simulink model "power_OLTCregtransformer"  (Simulink 6.0)
settings: Solver=ode23tb  StartTime=0.0  StopTime=120  MaxStep=1/60  RelTol=1e-4  AbsTol=1e-3
libraries: powerlib x75, powerlib_extras x18, simulink_extras x1
(part 3 of 3)

== system power_OLTCregtransformer/Three-Phase OLTC Regulating Transformer (Phasor Type)/Z & Voltage Ratio/Z Tap on winding 2 ==
  note: Tap changer on winding 2:
      | Z = Zw1  + Zw2*1/(1+NdU)^2 +  Ztmax*N*Nmax*(dU)^2/(1+NdU)^2
      | N1/N2= 1/(1+NdU)
      |
      | where :
      | Zw1   =  impedance of winding 1 (pu based on Pnom and V1nom)
      | Zw2   =  impedance of winding 2 (pu based on Pnom and V2nom)
      | Ztmax = impedance of tapped winding at maximum tap (Nmax)     (pu  based on  Pnom & Nmax*dU)
      | Zt =  impedance of tapped winding at tap N
      |      = Ztmax*N/Nmax*(Nmax.dU)^2 = Ztmax*N*Nmax*(dU)^2             (pu based on Pnom and V2nom)
  N : Inport  Port=1  LatchInput=off
  dU : Inport  Port=2  LatchInput=off
  Zw1 : Inport  Port=3  LatchInput=off
  Zw2 : Inport  Port=4  LatchInput=off
  Ztmax : Inport  Port=5  LatchInput=off
  Nmax : Inport  Port=6  LatchInput=off
  Enable : EnablePort
  Math Function1 : Math  Operator=reciprocal  SaturateOnIntegerOverflow=on
  Math Function2 : Math  Operator=square  SaturateOnIntegerOverflow=on
  Math Function5 : Math  Operator=square  SaturateOnIntegerOverflow=on
  Product1 : Product  SaturateOnIntegerOverflow=on
  Product2 : Product  Inputs=*/  SaturateOnIntegerOverflow=on
  Product3 : Product  Inputs=****  SaturateOnIntegerOverflow=on
  Product6 : Product  Inputs=*/  SaturateOnIntegerOverflow=on
  Psi1 : Constant
  Sum1 : Sum  Inputs=+++  SaturateOnIntegerOverflow=on
  Sum2 : Sum  SaturateOnIntegerOverflow=on
  Z : Outport
  N1/N2 : Outport  Port=2
  wires:
  Math Function1/1 -> N1/N2/1
  Product6/1 -> Sum1/1
  Product3/1 -> Product6/1  "Zt = Ztmax*N*Nmax*(dU)^2"
  Math Function2/1 -> Product6/2, Product2/2
  Zw2/1 -> Product2/1
  Product2/1 -> Sum1/2
  Sum1/1 -> Z/1
  Zw1/1 -> Sum1/3
  Psi1/1 -> Sum2/2
  Sum2/1 -> Math Function1/1, Math Function2/1  "1+NdU"
  N/1 -> Product1/1, Product3/3
  dU/1 -> Math Function5/1, Product1/2
  Product1/1 -> Sum2/1  "NdU"
  Ztmax/1 -> Product3/1
  Nmax/1 -> Product3/2
  Math Function5/1 -> Product3/4

== system power_OLTCregtransformer/Three-Phase OLTC Regulating Transformer/ OLTC Control/Monostable/Edge Detector ==
  note: Edge or Slope Detector
  note: Silvano Casoria
      | Power System Simulation Laboratory
      | IREQ, Hydro-Quebec
  In : Inport  Port=1  LatchInput=off
  Constant1 : Constant  Value=model
  Demux : Demux  Outputs=2
  Logical Operator1 : Logic  Operator=OR
  Memory : Memory  X0=ic  InheritSampleTime=on
  Multiport Switch : MultiPortSwitch  Inputs=3  SaturateOnIntegerOverflow=on
  NEGATIVE Edge : Subsystem  AncestorBlock=extra_sc/Edge/POSITIVE Edge  TreatAsAtomicUnit=on
  POSITIVE Edge : Subsystem  AncestorBlock=extra_sc/Delay_discrete/OFF Delay  TreatAsAtomicUnit=on
  either edge : Constant  Value=[1 1]
  neg. edge : Constant  Value=[0 1]
  pos. edge : Constant  Value=[1 0]
  Out : Outport
  wires:
  either edge/1 -> Multiport Switch/4
  Demux/2 -> NEGATIVE Edge/Enable
  Demux/1 -> POSITIVE Edge/Enable
  Multiport Switch/1 -> Demux/1
  Constant1/1 -> Multiport Switch/1
  neg. edge/1 -> Multiport Switch/3
  pos. edge/1 -> Multiport Switch/2
  In/1 -> Memory/1, NEGATIVE Edge/1(IN), POSITIVE Edge/1(IN)
  Memory/1 -> NEGATIVE Edge/2(IN previous), POSITIVE Edge/2(IN previous)
  POSITIVE Edge/1(OUT) -> Logical Operator1/1
  NEGATIVE Edge/1(OUT) -> Logical Operator1/2
  Logical Operator1/1 -> Out/1

== system power_OLTCregtransformer/Three-Phase OLTC Regulating Transformer/ OLTC Control/Tap Changer Control/Determine tap positon ==
  NewTap : Inport  Port=1  LatchInput=off
  Trigger : TriggerPort
  Memory : Memory  Orientation=left  X0=InitialPosition  InheritSampleTime=on
  Saturation : Saturate  UpperLimit=MinMaxTap(2)  LowerLimit=MinMaxTap(1)
  Sum : Sum  Inputs=|++  SaturateOnIntegerOverflow=on
  TapNo : Outport  InitialOutput=InitialPosition
  wires:
  NewTap/1 -> Sum/1
  Sum/1 -> Saturation/1
  Memory/1 -> Sum/2
  Saturation/1 -> TapNo/1, Memory/1

== system power_OLTCregtransformer/Three-Phase OLTC Regulating Transformer (Phasor Type)/ Currents /dq0 model of 3-ph RL branch/Negative-sequence dq0 model of a 3-phase series R-L branch ==
  note: Using Laplace transform and per unit (pu) quantities :
  note: d-q axis model of a 3-phase series R-L branch
  note: Id = [ w / ( L * s ) ] * [ Vd1 - Vd2 - ( R * Id ) + ( L * Iq ) ]
  note: Iq = [ w / ( L * s ) ] * [ Vq1 - Vq2 - ( R * Iq ) - ( L * Id ) ]
  note: where w = 2*pi*Fnom (Hz)
  note: Vd1 - Vd2 = [ R * Id ] - [ L* w * Iq ] + [ L * d/dt (Id) ]
  note: o--------| R |---| L |-------o
  note: V1
  note: V2
  note: I --->
  note: ==========================================================================================
  note: Vq1 - Vq2 = [ R * Iq ] + [ L* w * Id ] + [ L * d/dt (Iq) ]
  note: where w = 2*pi*Fnom (Hz)
  Vdq1 : Inport  Port=1  LatchInput=off
  Vdq2 : Inport  Port=2  LatchInput=off
  R_L : Inport  Port=3  LatchInput=off
  Demux3 : Demux  Outputs=2
  Integrator : Integrator
  Product : Product  SaturateOnIntegerOverflow=on
  Product1 : Product  SaturateOnIntegerOverflow=on
  Product2 : Product  Inputs=*/  SaturateOnIntegerOverflow=on
  R_choke2 : Gain  Gain=[1 -1]  SaturateOnIntegerOverflow=on
  R_choke3 : Gain  Gain=w  SaturateOnIntegerOverflow=on
  Selector : Selector  Elements=[2 1]  InputPortWidth=2
  Sum : Sum  Inputs=+--+  SaturateOnIntegerOverflow=on
  idIq : Outport
  wires:
  Vdq1/1 -> Sum/1
  Vdq2/1 -> Sum/2
  Product/1 -> Sum/3
  R_choke2/1 -> Sum/4
  Product1/1 -> R_choke2/1
  Sum/1 -> R_choke3/1
  Integrator/1 -> idIq/1, Selector/1, Product/1
  Selector/1 -> Product1/1
  R_choke3/1 -> Product2/1
  Product2/1 -> Integrator/1
  R_L/1 -> Demux3/1
  Demux3/2 -> Product2/2, Product1/2
  Demux3/1 -> Product/2

== system power_OLTCregtransformer/Three-Phase OLTC Regulating Transformer (Phasor Type)/ Currents /dq0 model of 3-ph RL branch/Positive-sequence dq0 model of a 3-phase series R-L branch ==
  note: where w = 2*pi*Fnom (Hz)
  note: Vq1 - Vq2 = [ R * Iq ] + [ L* w * Id ] + [ L * d/dt (Iq) ]
  note: ==========================================================================================
  note: I --->
  note: V2
  note: V1
  note: o--------| R |---| L |-------o
  note: Vd1 - Vd2 = [ R * Id ] - [ L* w * Iq ] + [ L * d/dt (Id) ]
  note: where w = 2*pi*Fnom (Hz)
  note: Iq = [ w / ( L * s ) ] * [ Vq1 - Vq2 - ( R * Iq ) - ( L * Id ) ]
  note: Id = [ w / ( L * s ) ] * [ Vd1 - Vd2 - ( R * Id ) + ( L * Iq ) ]
  note: d-q axis model of a 3-phase series R-L branch
  note: Using Laplace transform and per unit (pu) quantities :
  Vdq1 : Inport  Port=1  LatchInput=off
  Vdq2 : Inport  Port=2  LatchInput=off
  R_L : Inport  Port=3  LatchInput=off
  Demux3 : Demux  Outputs=2
  Integrator : Integrator  InitialCondition="[I21_init_real   I21_init_imag]"
  Product : Product  SaturateOnIntegerOverflow=on
  Product1 : Product  SaturateOnIntegerOverflow=on
  Product2 : Product  Inputs=*/  SaturateOnIntegerOverflow=on
  R_choke2 : Gain  Gain=[1 -1]  SaturateOnIntegerOverflow=on
  R_choke3 : Gain  Gain=w  SaturateOnIntegerOverflow=on
  Selector : Selector  Elements=[2 1]  InputPortWidth=2
  Sum : Sum  Inputs=+--+  SaturateOnIntegerOverflow=on
  idIq : Outport
  wires:
  Demux3/1 -> Product/2
  Demux3/2 -> Product1/2, Product2/2
  R_L/1 -> Demux3/1
  Product2/1 -> Integrator/1
  R_choke3/1 -> Product2/1
  Selector/1 -> Product1/1
  Integrator/1 -> Product/1, Selector/1, idIq/1
  Sum/1 -> R_choke3/1
  Product1/1 -> R_choke2/1
  R_choke2/1 -> Sum/4
  Product/1 -> Sum/3
  Vdq2/1 -> Sum/2
  Vdq1/1 -> Sum/1

== system power_OLTCregtransformer/Three-Phase OLTC Regulating Transformer (Phasor Type)/ Currents /dq0 model of 3-ph RL branch/Zero-sequence dq0 model of a 3-phase series R-L branch ==
  note: where w = 2*pi*Fnom (Hz)
  note: Vq1 - Vq2 = [ R * Iq ] + [ L* w * Id ] + [ L * d/dt (Iq) ]
  note: ==========================================================================================
  note: I --->
  note: V2
  note: V1
  note: o--------| R |---| L |-------o
  note: Vd1 - Vd2 = [ R * Id ] - [ L* w * Iq ] + [ L * d/dt (Id) ]
  note: where w = 2*pi*Fnom (Hz)
  note: Iq = [ w / ( L * s ) ] * [ Vq1 - Vq2 - ( R * Iq ) - ( L * Id ) ]
  note: Id = [ w / ( L * s ) ] * [ Vd1 - Vd2 - ( R * Id ) + ( L * Iq ) ]
  note: d-q axis model of a 3-phase series R-L branch
  note: Using Laplace transform and per unit (pu) quantities :
  Vdq1 : Inport  Port=1  LatchInput=off
  Vdq2 : Inport  Port=2  LatchInput=off
  R_L : Inport  Port=3  LatchInput=off
  Demux3 : Demux  Outputs=2
  Integrator : Integrator
  Product : Product  SaturateOnIntegerOverflow=on
  Product1 : Product  SaturateOnIntegerOverflow=on
  Product2 : Product  Inputs=*/  SaturateOnIntegerOverflow=on
  R_choke2 : Gain  Gain=[1 -1]  SaturateOnIntegerOverflow=on
  R_choke3 : Gain  Gain=w  SaturateOnIntegerOverflow=on
  Selector : Selector  Elements=[2 1]  InputPortWidth=2
  Sum : Sum  Inputs=+--+  SaturateOnIntegerOverflow=on
  idIq : Outport
  wires:
  Demux3/1 -> Product/2
  Demux3/2 -> Product1/2, Product2/2
  R_L/1 -> Demux3/1
  Product2/1 -> Integrator/1
  R_choke3/1 -> Product2/1
  Selector/1 -> Product1/1
  Integrator/1 -> Product/1, Selector/1, idIq/1
  Sum/1 -> R_choke3/1
  Product1/1 -> R_choke2/1
  R_choke2/1 -> Sum/4
  Product/1 -> Sum/3
  Vdq2/1 -> Sum/2
  Vdq1/1 -> Sum/1

== system power_OLTCregtransformer/Three-Phase OLTC Regulating Transformer/ OLTC Control/Monostable/Edge Detector/NEGATIVE Edge ==
  IN : Inport  Port=1  LatchInput=off
  IN previous : Inport  Port=2  LatchInput=off
  Enable : EnablePort
  Relational Operator1 : RelationalOperator  Operator=>  InputSameDT=on
  OUT : Outport
  wires:
  IN/1 -> Relational Operator1/2
  IN previous/1 -> Relational Operator1/1
  Relational Operator1/1 -> OUT/1

== system power_OLTCregtransformer/Three-Phase OLTC Regulating Transformer/ OLTC Control/Monostable/Edge Detector/POSITIVE Edge ==
  IN : Inport  Port=1  LatchInput=off
  IN previous : Inport  Port=2  LatchInput=off
  Enable : EnablePort
  Relational Operator1 : RelationalOperator  Operator=>  InputSameDT=on
  OUT : Outport
  wires:
  IN/1 -> Relational Operator1/1
  IN previous/1 -> Relational Operator1/2
  Relational Operator1/1 -> OUT/1
